simulink model "nms_model"  (Simulink 7.5)
settings: Solver=ode15s  StartTime=0.0  StopTime=60  FixedStep=1e-3  MaxStep=ts_max  RelTol=1e-3  AbsTol=1e-4
InitFcn:
  | nms_model_MechInit
  | nms_model_ControlInit
values from neighbouring files (symbols this model uses):
  c = 0.05    [muscleParams.m]    (also in nms_model_MechInit.m)
  c_jointstop = 0.3 / (pi/180)    (= 17.1887338539)    [muscleParams.m]    (also in nms_model_MechInit.m)
  D12_F = 0.16    [nms_model_MechInit.m]
  D12_S = L_S    (= 0.5)    [nms_model_MechInit.m]
  D12_T = L_T    (= 0.5)    [nms_model_MechInit.m]
  D13_F = 0.20    (= 0.2)    [nms_model_MechInit.m]
  D1G_F = 0.14    [nms_model_MechInit.m]
  D1G_HAT = 0.35    [nms_model_MechInit.m]
  D1G_S = 0.3    [nms_model_MechInit.m]
  D1G_T = 0.3    [nms_model_MechInit.m]
  DeltaThRef = 5e-3    (= 0.005)    [nms_model_MechInit.m]
  eref = 0.04    [muscleParams.m]    (also in nms_model_MechInit.m)
  FmaxGAS = 1500    [nms_model_MechInit.m]
  FmaxGLU = 1500    [nms_model_MechInit.m]
  FmaxHAM = 3000    [nms_model_MechInit.m]
  FmaxHFL = 2000    [nms_model_MechInit.m]
  FmaxSOL = 4000    [nms_model_MechInit.m]
  FmaxTA = 800    [nms_model_MechInit.m]
  FmaxVAS = 300    [muscleParams.m]    (also in nms_model_MechInit.m = 6000)
  GainDeltaTheta = 2 /100*180/pi    (= 1.14591559026)    [nms_model_ControlInit.m]
  GainGAS = 1.1/FmaxGAS    [nms_model_ControlInit.m]
  GainGLU = 0.5/FmaxGLU    [nms_model_ControlInit.m]
  GainHAM = 0.65/FmaxHAM    [nms_model_ControlInit.m]
  GainHAMHFL = 4    [nms_model_ControlInit.m]
  GainHFL = 0.5    [nms_model_ControlInit.m]
  GainKneOverExt = 2    [nms_model_ControlInit.m]
  GainSOL = 1.2/FmaxSOL    [nms_model_ControlInit.m]
  GainSOLTA = 0.4/FmaxSOL    [nms_model_ControlInit.m]
  GainTA = 1.1    [nms_model_ControlInit.m]
  GainVAS = 1.2/FmaxVAS    [nms_model_ControlInit.m]
  In_F = 0.005    [nms_model_MechInit.m]
  In_HAT = 3    [nms_model_MechInit.m]
  In_S = 0.05    [nms_model_MechInit.m]
  In_T = 0.15    [nms_model_MechInit.m]
  K = 5    [muscleParams.m]    (also in nms_model_MechInit.m)
  k_gx = (2*(m_F+m_S+m_T)+m_HAT)*g/0.1    (= 7848)    [nms_model_MechInit.m]
  k_gy = (2*(m_F+m_S+m_T)+m_HAT)*g/0.01    (= 78480)    [nms_model_MechInit.m]
  k_pressure = m_HAT * 9.81 / DeltaThRef    (= 104967)    [nms_model_MechInit.m]
  K_swing = 0.25    [nms_model_ControlInit.m]
  KneePh23Offset = 170*pi/180    (= 2.96705972839)    [nms_model_ControlInit.m]
  LceOffsetHAM = 0.85    [nms_model_ControlInit.m]
  LceOffsetHFL = 0.65    [nms_model_ControlInit.m]
  LceOffsetTA = 1-0.5*w    [nms_model_ControlInit.m]
  LongDelay = 0.020    (= 0.02)    [nms_model_ControlInit.m]
  loptGAS = 0.05    [nms_model_MechInit.m]
  loptGLU = 0.11    [nms_model_MechInit.m]
  loptHAM = 0.10    (= 0.1)    [nms_model_MechInit.m]
  loptHFL = 0.11    [nms_model_MechInit.m]
  loptSOL = 0.04    [nms_model_MechInit.m]
  loptTA = 0.06    [nms_model_MechInit.m]
  loptVAS = 0.13    [muscleParams.m]    (also in nms_model_MechInit.m = 0.08)
  lslackGAS = 0.40    (= 0.4)    [nms_model_MechInit.m]
  lslackGLU = 0.13    [nms_model_MechInit.m]
  lslackHAM = 0.31    [nms_model_MechInit.m]
  lslackHFL = 0.10    (= 0.1)    [nms_model_MechInit.m]
  lslackSOL = 0.26    [nms_model_MechInit.m]
  lslackTA = 0.24    [nms_model_MechInit.m]
  lslackVAS = 0.23    [muscleParams.m]    (also in nms_model_MechInit.m)
  m_F = 1.25    [nms_model_MechInit.m]
  m_HAT = 53.5    [nms_model_MechInit.m]
  m_S = 3.5    [nms_model_MechInit.m]
  m_T = 8.5    [nms_model_MechInit.m]
  MidDelay = 0.010    (= 0.01)    [nms_model_ControlInit.m]
  mu_slide = 0.8    [nms_model_MechInit.m]
  mu_stick = 0.9    [nms_model_MechInit.m]
  N = 1.5    [muscleParams.m]    (also in nms_model_MechInit.m)
  phi12_LowLimit = 70*pi/180    (= 1.2217304764)    [nms_model_MechInit.m]
  phi12_UpLimit = 180*pi/180    (= 3.14159265359)    [muscleParams.m]    (also in nms_model_MechInit.m = 2.26892802759)
  phi23_UpLimit = 159*pi/180    (= 2.77507351067)    [muscleParams.m]    (also in nms_model_MechInit.m = 3.05432619099)
  phi34_UpLimit = 230*pi/180    (= 4.01425727959)    [nms_model_MechInit.m]
  phimaxGASa = 110*pi/180    (= 1.91986217719)    [nms_model_MechInit.m]
  phimaxGASk = 140*pi/180    (= 2.44346095279)    [nms_model_MechInit.m]
  phimaxHAMk = 180*pi/180    (= 3.14159265359)    [nms_model_MechInit.m]
  phimaxSOL = 110*pi/180    (= 1.91986217719)    [nms_model_MechInit.m]
  phimaxTA = 80*pi/180    (= 1.3962634016)    [nms_model_MechInit.m]
  phimaxVAS = 90*pi/180    (= 1.57079632679)    [muscleParams.m]    (also in nms_model_MechInit.m = 2.87979326579)
  phirefGASa = 80*pi/180    (= 1.3962634016)    [nms_model_MechInit.m]
  phirefGASk = 165*pi/180    (= 2.87979326579)    [nms_model_MechInit.m]
  phirefGLU = 150*pi/180    (= 2.61799387799)    [nms_model_MechInit.m]
  phirefHAMh = 155*pi/180    (= 2.70526034059)    [nms_model_MechInit.m]
  phirefHAMk = 180*pi/180    (= 3.14159265359)    [nms_model_MechInit.m]
  phirefHFL = 180*pi/180    (= 3.14159265359)    [nms_model_MechInit.m]
  phirefSOL = 80*pi/180    (= 1.3962634016)    [nms_model_MechInit.m]
  phirefTA = 110*pi/180    (= 1.91986217719)    [nms_model_MechInit.m]
  phirefVAS = 60*pi/180    (= 1.0471975512)    [muscleParams.m]    (also in nms_model_MechInit.m = 2.18166156499)
  PosGainGG = 1/(30*pi/180)    (= 1.9098593171)    [nms_model_ControlInit.m]
  PreStimGAS = 0.01    [nms_model_ControlInit.m]
  PreStimGG = 0.05    [nms_model_ControlInit.m]
  PreStimGLU = 0.01    [nms_model_ControlInit.m]
  PreStimHAM = 0.01    [nms_model_ControlInit.m]
  PreStimHFL = 0.01    [nms_model_ControlInit.m]
  PreStimSOL = 0.01    [nms_model_ControlInit.m]
  PreStimTA = 0.01    [nms_model_ControlInit.m]
  PreStimVAS = 0.08    [nms_model_ControlInit.m]
  rGASa = 0.05    [nms_model_MechInit.m]
  rGASk = 0.05    [nms_model_MechInit.m]
  rGLU = 0.10    (= 0.1)    [nms_model_MechInit.m]
  rHAMh = 0.08    [nms_model_MechInit.m]
  rHAMk = 0.05    [nms_model_MechInit.m]
  rHFL = 0.10    (= 0.1)    [nms_model_MechInit.m]
  rhoGASa = 0.7    [nms_model_MechInit.m]
  rhoGASk = 0.7    [nms_model_MechInit.m]
  rhoGLU = 0.5    [nms_model_MechInit.m]
  rhoHAMh = 0.7    [nms_model_MechInit.m]
  rhoHAMk = 0.7    [nms_model_MechInit.m]
  rhoHFL = 0.5    [nms_model_MechInit.m]
  rhoSOL = 0.5    [nms_model_MechInit.m]
  rhoTA = 0.7    [nms_model_MechInit.m]
  rhoVAS = 3    [muscleParams.m]    (also in nms_model_MechInit.m = 0.7)
  rSOL = 0.05    [nms_model_MechInit.m]
  rTA = 0.04    [nms_model_MechInit.m]
  rVAS = 0.03    [muscleParams.m]    (also in nms_model_MechInit.m = 0.06)
  s = orProblemSendCommand(['LoadIKFastSolver robot Translation3D'],probid)    [init.m]
  ShortDelay = 0.005    [nms_model_ControlInit.m]
  SpeedGainGG = 0.2    [nms_model_ControlInit.m]
  tau = 0.01    [muscleParams.m]    (also in nms_model_MechInit.m)
  Theta0 = 6*pi/180    (= 0.10471975512)    [nms_model_ControlInit.m]
  ThPos = 4/5    (= 0.8)    [nms_model_MechInit.m]
  v_gx_max = 0.03    [nms_model_MechInit.m]
  v_gy_max = 0.03    [nms_model_MechInit.m]
  ... (+11 more)
undefined symbols (not defined in the file or in its folder): sgn
libraries: mblibv1 x60, simulink x22, simulink_extras x20
(part 5 of 9)

== system nms_model/Muscle Actuation Layer/R TA ==
  note: Excitation Contraction Coupling
  note: Tibialis Anterior Muscle-Tendon Dynamics
  STIM : Inport  OutDataType=sfix(16)  OutScaling=2^0
  lmtc [m] : Inport  Port=2  OutDataType=sfix(16)  OutScaling=2^0
  1 : Product  Inputs=**  OutDataType=sfix(16)  OutScaling=2^0  SaturateOnIntegerOverflow=on  InputSameDT=on  OutDataTypeStr=Inherit: Same as first input
  1/lslack : Gain  Gain=1/lslackTA  ParameterDataType=sfix(16)  ParameterScaling=2^0  OutDataType=sfix(16)  OutScaling=2^0  SaturateOnIntegerOverflow=on  OutDataTypeStr=Inherit: Same as input  ParamDataTypeStr=Inherit: Same as input
  BE force-length relation : Subsystem
  CE force-length relation : Subsystem
  CE inverse  force-velocity relation : Subsystem
  Constant : Constant  Value=lslackTA  OutDataType=sfix(16)  OutScaling=2^0
  ECC TransferFcn : simulink_extras/Additional Linear/Transfer Fcn (with initial outputs)  SystemSampleTime=-1  N=[1]  D="[tau  1]"  Y0=preA  U0=0
      settings: AttributesFormatString=pre-activation: %<Y0>
  Fmax : Gain  Gain=FmaxTA  ParameterDataType=sfix(16)  ParameterScaling=2^0  OutDataType=sfix(16)  OutScaling=2^0  SaturateOnIntegerOverflow=on  OutDataTypeStr=Inherit: Same as input  ParamDataTypeStr=Inherit: Same as input
  Fv = Fse / (A*Fce) : Product  Inputs=*/  OutDataType=sfix(16)  OutScaling=2^0  SaturateOnIntegerOverflow=on  InputSameDT=on  OutDataTypeStr=Inherit: Same as first input
  Integrator : Integrator  InitialConditionSource=external  LowerSaturationLimit=0.05
  PE force-length relation : Subsystem
  SE force-length relation : Subsystem
  Sum : Sum  Inputs=|+-  OutDataType=sfix(16)  OutScaling=2^0  SaturateOnIntegerOverflow=on  InputSameDT=on  OutDataTypeStr=Inherit: Same as first input
  Sum2 : Sum  Inputs=|-+  OutDataType=sfix(16)  OutScaling=2^0  SaturateOnIntegerOverflow=on  InputSameDT=on  OutDataTypeStr=Inherit: Same as first input
  Sum3 : Sum  OutDataType=sfix(16)  OutScaling=2^0  SaturateOnIntegerOverflow=on  InputSameDT=on  OutDataTypeStr=Inherit: Same as first input
  Sum4 : Sum  OutDataType=sfix(16)  OutScaling=2^0  SaturateOnIntegerOverflow=on  InputSameDT=on  OutDataTypeStr=Inherit: Same as first input
  lce/lopt : Gain  Gain=1/loptTA  ParameterDataType=sfix(16)  ParameterScaling=2^0  OutDataType=sfix(16)  OutScaling=2^0  SaturateOnIntegerOverflow=on  OutDataTypeStr=Inherit: Same as input  ParamDataTypeStr=Inherit: Same as input
  vmax*lopt : Gain  Gain=vmaxTA*loptTA  ParameterDataType=sfix(16)  ParameterScaling=2^0  OutDataType=sfix(16)  OutScaling=2^0  SaturateOnIntegerOverflow=on  OutDataTypeStr=Inherit: Same as input  ParamDataTypeStr=Inherit: Same as input
  Fmtc : Outport  OutDataType=sfix(16)  OutScaling=2^0  InitialOutput=0
  Lce : Outport  Port=2  OutDataType=sfix(16)  OutScaling=2^0  InitialOutput=0
  Vce : Outport  Port=3  OutDataType=sfix(16)  OutScaling=2^0  InitialOutput=0
  Lse : Outport  Port=4  OutDataType=sfix(16)  OutScaling=2^0  InitialOutput=0
  A : Outport  Port=5  OutDataType=sfix(16)  OutScaling=2^0  InitialOutput=0
  wires:
  CE inverse  force-velocity relation/1(v[vmax]) -> vmax*lopt/1
  Sum3/1 -> Fv = Fse / (A*Fce)/2
  BE force-length relation/1(fbe [Fmax]) -> Sum4/2
  1/1 -> Sum3/2
  PE force-length relation/1(fpe [Fmax]) -> Sum3/1
  Sum4/1 -> Fv = Fse / (A*Fce)/1
  CE force-length relation/1(fce [Fmax]) -> 1/1
  Constant/1 -> Sum2/1
  Sum2/1 -> Integrator/2
  SE force-length relation/1(fse [Fmax]) -> Sum4/1, Fmax/1
  1/lslack/1 -> SE force-length relation/1(lse [lslack])
  Fmax/1 -> Fmtc/1  "Fmtc"
  lmtc [m]/1 -> Sum/1, Sum2/2  "lmtc"
  vmax*lopt/1 -> Integrator/1, Vce/1  "vce"
  Fv = Fse / (A*Fce)/1 -> CE inverse  force-velocity relation/1(Fv[Fmax])  "fv"
  lce/lopt/1 -> PE force-length relation/1(lce [lopt]), BE force-length relation/1(lce [lopt]), CE force-length relation/1(lce [lopt])
  Sum/1 -> Lse/1, 1/lslack/1  "lse"
  Integrator/1 -> lce/lopt/1, Sum/2, Lce/1  "lce"
  STIM/1 -> ECC TransferFcn/1
  ECC TransferFcn/1 -> 1/2, A/1

== system nms_model/Muscle Actuation Layer/R TA Link ==
  note: Muscle Length and Moment Arm
  phi12 [rad] : Inport  OutDataType=sfix(16)  OutScaling=2^0
  Constant : Constant  Value=lslackTA+loptTA  OutDataType=sfix(16)  OutScaling=2^0
  Constant2 : Constant  Value=phirefTA  OutDataType=sfix(16)  OutScaling=2^0
  Constant3 : Constant  Value=phimaxTA  OutDataType=sfix(16)  OutScaling=2^0
  Demux : Demux  Outputs=2
  Gain2 : Gain  Gain=rTA  ParameterDataType=sfix(16)  ParameterScaling=2^0  OutDataType=sfix(16)  OutScaling=2^0
  Gain4 : Gain  Gain=rhoTA  ParameterDataType=sfix(16)  ParameterScaling=2^0  OutDataType=sfix(16)  OutScaling=2^0
  Mux : Mux  Inputs=2
  Sum2 : Sum  Inputs=|+-  OutDataType=sfix(16)  OutScaling=2^0
  Sum3 : Sum  Inputs=-+|  OutDataType=sfix(16)  OutScaling=2^0
  Sum4 : Sum  Inputs=+-  OutDataType=sfix(16)  OutScaling=2^0
  Sum5 : Sum  Inputs=|+-  OutDataType=sfix(16)  OutScaling=2^0
  length change term : Trigonometry
  offset correction term : Trigonometry
  variable lever term : Trigonometry  Operator=cos
  lmtc [m] : Outport  OutDataType=sfix(16)  OutScaling=2^0
  lever [m] : Outport  Port=2  OutDataType=sfix(16)  OutScaling=2^0
  wires:
  phi12 [rad]/1 -> Sum3/2
  Sum3/1 -> variable lever term/1, length change term/1
  Constant3/1 -> Sum3/1, Sum2/2
  Sum2/1 -> offset correction term/1
  Constant2/1 -> Sum2/1
  length change term/1 -> Sum4/2
  offset correction term/1 -> Sum4/1
  Sum4/1 -> Mux/1
  Constant/1 -> Sum5/1
  Sum5/1 -> lmtc [m]/1
  Gain4/1 -> Sum5/2
  variable lever term/1 -> Mux/2
  Mux/1 -> Gain2/1
  Gain2/1 -> Demux/1
  Demux/1 -> Gain4/1
  Demux/2 -> lever [m]/1

== system nms_model/Muscle Actuation Layer/R VAS ==
  note: VASTI Muscle-Tendon Dynamics
  note: Excitation Contraction Coupling
  STIM : Inport  OutDataType=sfix(16)  OutScaling=2^0
  lmtc [m] : Inport  Port=2  OutDataType=sfix(16)  OutScaling=2^0
  1 : Product  Inputs=**  OutDataType=sfix(16)  OutScaling=2^0  SaturateOnIntegerOverflow=on  InputSameDT=on  OutDataTypeStr=Inherit: Same as first input
  1/lslack : Gain  Gain=1/lslackVAS  ParameterDataType=sfix(16)  ParameterScaling=2^0  OutDataType=sfix(16)  OutScaling=2^0  SaturateOnIntegerOverflow=on  OutDataTypeStr=Inherit: Same as input  ParamDataTypeStr=Inherit: Same as input
  BE force-length relation : Subsystem
  CE force-length relation : Subsystem
  CE inverse  force-velocity relation : Subsystem
  Constant : Constant  Value=lslackVAS  OutDataType=sfix(16)  OutScaling=2^0
  ECC TransferFcn : simulink_extras/Additional Linear/Transfer Fcn (with initial outputs)  SystemSampleTime=-1  N=[1]  D="[tau  1]"  Y0=preA  U0=0
      settings: AttributesFormatString=pre-activation: %<Y0>
  Fmax : Gain  Gain=FmaxVAS  ParameterDataType=sfix(16)  ParameterScaling=2^0  OutDataType=sfix(16)  OutScaling=2^0  SaturateOnIntegerOverflow=on  OutDataTypeStr=Inherit: Same as input  ParamDataTypeStr=Inherit: Same as input
  Fv = Fse / (A*Fce) : Product  Inputs=*/  OutDataType=sfix(16)  OutScaling=2^0  SaturateOnIntegerOverflow=on  InputSameDT=on  OutDataTypeStr=Inherit: Same as first input
  Integrator : Integrator  InitialConditionSource=external  LowerSaturationLimit=0.05
  PE force-length relation : Subsystem
  SE force-length relation : Subsystem
  Sum : Sum  Inputs=|+-  OutDataType=sfix(16)  OutScaling=2^0  SaturateOnIntegerOverflow=on  InputSameDT=on  OutDataTypeStr=Inherit: Same as first input
  Sum2 : Sum  Inputs=|-+  OutDataType=sfix(16)  OutScaling=2^0  SaturateOnIntegerOverflow=on  InputSameDT=on  OutDataTypeStr=Inherit: Same as first input
  Sum3 : Sum  OutDataType=sfix(16)  OutScaling=2^0  SaturateOnIntegerOverflow=on  InputSameDT=on  OutDataTypeStr=Inherit: Same as first input
  Sum4 : Sum  OutDataType=sfix(16)  OutScaling=2^0  SaturateOnIntegerOverflow=on  InputSameDT=on  OutDataTypeStr=Inherit: Same as first input
  lce/lopt : Gain  Gain=1/loptVAS  ParameterDataType=sfix(16)  ParameterScaling=2^0  OutDataType=sfix(16)  OutScaling=2^0  SaturateOnIntegerOverflow=on  OutDataTypeStr=Inherit: Same as input  ParamDataTypeStr=Inherit: Same as input
  vmax*lopt : Gain  Gain=vmaxVAS*loptVAS  ParameterDataType=sfix(16)  ParameterScaling=2^0  OutDataType=sfix(16)  OutScaling=2^0  SaturateOnIntegerOverflow=on  OutDataTypeStr=Inherit: Same as input  ParamDataTypeStr=Inherit: Same as input
  Fmtc : Outport  OutDataType=sfix(16)  OutScaling=2^0  InitialOutput=0
  Lce : Outport  Port=2  OutDataType=sfix(16)  OutScaling=2^0  InitialOutput=0
  Vce : Outport  Port=3  OutDataType=sfix(16)  OutScaling=2^0  InitialOutput=0
  Lse : Outport  Port=4  OutDataType=sfix(16)  OutScaling=2^0  InitialOutput=0
  A : Outport  Port=5  OutDataType=sfix(16)  OutScaling=2^0  InitialOutput=0
  wires:
  Integrator/1 -> Sum/2, lce/lopt/1, Lce/1  "lce"
  Sum/1 -> 1/lslack/1, Lse/1  "lse"
  lce/lopt/1 -> CE force-length relation/1(lce [lopt]), BE force-length relation/1(lce [lopt]), PE force-length relation/1(lce [lopt])
  Fv = Fse / (A*Fce)/1 -> CE inverse  force-velocity relation/1(Fv[Fmax])  "fv"
  vmax*lopt/1 -> Integrator/1, Vce/1  "vce"
  lmtc [m]/1 -> Sum2/2, Sum/1  "lmtc"
  Fmax/1 -> Fmtc/1  "Fmtc"
  1/lslack/1 -> SE force-length relation/1(lse [lslack])
  SE force-length relation/1(fse [Fmax]) -> Fmax/1, Sum4/1
  Sum2/1 -> Integrator/2
  Constant/1 -> Sum2/1
  CE force-length relation/1(fce [Fmax]) -> 1/1
  Sum4/1 -> Fv = Fse / (A*Fce)/1
  PE force-length relation/1(fpe [Fmax]) -> Sum3/1
  1/1 -> Sum3/2
  BE force-length relation/1(fbe [Fmax]) -> Sum4/2
  Sum3/1 -> Fv = Fse / (A*Fce)/2
  CE inverse  force-velocity relation/1(v[vmax]) -> vmax*lopt/1
  STIM/1 -> ECC TransferFcn/1
  ECC TransferFcn/1 -> 1/2, A/1

== system nms_model/Muscle Actuation Layer/R VAS Link ==
  note: Muscle Length and Moment Arm
  phi23 [rad] : Inport  OutDataType=sfix(16)  OutScaling=2^0
  Constant : Constant  Value=lslackVAS+loptVAS  OutDataType=sfix(16)  OutScaling=2^0
  Constant2 : Constant  Value=phirefVAS  OutDataType=sfix(16)  OutScaling=2^0
  Constant3 : Constant  Value=phimaxVAS  OutDataType=sfix(16)  OutScaling=2^0
  Demux : Demux  Outputs=2
  Gain2 : Gain  Gain=rVAS  ParameterDataType=sfix(16)  ParameterScaling=2^0  OutDataType=sfix(16)  OutScaling=2^0
  Gain4 : Gain  Gain=rhoVAS  ParameterDataType=sfix(16)  ParameterScaling=2^0  OutDataType=sfix(16)  OutScaling=2^0
  Mux : Mux  Inputs=2
  Sum2 : Sum  Inputs=|+-  OutDataType=sfix(16)  OutScaling=2^0
  Sum3 : Sum  Inputs=-+|  OutDataType=sfix(16)  OutScaling=2^0
  Sum4 : Sum  Inputs=+-  OutDataType=sfix(16)  OutScaling=2^0
  Sum5 : Sum  Inputs=|++  OutDataType=sfix(16)  OutScaling=2^0
  length change term : Trigonometry
  offset correction term : Trigonometry
  variable lever term : Trigonometry  Operator=cos
  lmtu [m] : Outport  OutDataType=sfix(16)  OutScaling=2^0
  lever [m] : Outport  Port=2  OutDataType=sfix(16)  OutScaling=2^0
  wires:
  phi23 [rad]/1 -> Sum3/2
  Sum3/1 -> variable lever term/1, length change term/1
  Constant3/1 -> Sum3/1, Sum2/2
  Sum2/1 -> offset correction term/1
  Constant2/1 -> Sum2/1
  length change term/1 -> Sum4/2
  offset correction term/1 -> Sum4/1
  Sum4/1 -> Mux/1
  Constant/1 -> Sum5/1
  Sum5/1 -> lmtu [m]/1
  Gain4/1 -> Sum5/2
  variable lever term/1 -> Mux/2
  Mux/1 -> Gain2/1
  Gain2/1 -> Demux/1
  Demux/1 -> Gain4/1
  Demux/2 -> lever [m]/1

== system nms_model/Neural Control Layer/Cross Influence Detection ==
  note: right leg is leading
  note: left leg is leading
  note: Double Support Cross Influences
  LStance : Inport  OutDataType=sfix(16)  OutScaling=2^0
  RStance : Inport  Port=2  OutDataType=sfix(16)  OutScaling=2^0
  DSup ends : HitCross  HitCrossingOffset=0.5  HitCrossingDirection=falling  ZeroCross=off
  Double Support? : Logic  AllPortsSameDT=off
  Double Support?1 : Logic  AllPortsSameDT=off
  Double Support?4 : Logic  AllPortsSameDT=off
  Flight? : Logic  Operator=NOR  AllPortsSameDT=off
  LLeg starts DSup : HitCross  HitCrossingOffset=0.5  HitCrossingDirection=rising  ZeroCross=off
  Memory : Memory
  Memory3 : Memory
  RLeg starts DSup : HitCross  HitCrossingOffset=0.5  HitCrossingDirection=rising  ZeroCross=off
  S-R Flip-Flop : simulink_extras/Flip Flops/S-R Flip-Flop  SystemSampleTime=-1  initial_condition=0
  S-R Flip-Flop1 : simulink_extras/Flip Flops/S-R Flip-Flop  SystemSampleTime=-1  initial_condition=0
  Terminator1 : Terminator
  Terminator2 : Terminator
  RonL : Outport  OutDataType=sfix(16)  OutScaling=2^0
  Flight : Outport  Port=2  OutDataType=sfix(16)  OutScaling=2^0
  LonR : Outport  Port=3  OutDataType=sfix(16)  OutScaling=2^0
  wires:
  S-R Flip-Flop/2 -> Terminator1/1
  Double Support?/1 -> DSup ends/1, Double Support?1/1, Double Support?4/2
  S-R Flip-Flop/1 -> LonR/1
  S-R Flip-Flop1/2 -> Terminator2/1
  LStance/1 -> Memory3/1, Double Support?/1, Flight?/1
  RStance/1 -> Memory/1, Double Support?/2, Flight?/2
  S-R Flip-Flop1/1 -> RonL/1
  Memory/1 -> RLeg starts DSup/1
  RLeg starts DSup/1 -> Double Support?1/2
  Double Support?1/1 -> S-R Flip-Flop1/1
  Memory3/1 -> LLeg starts DSup/1
  LLeg starts DSup/1 -> Double Support?4/1
  Double Support?4/1 -> S-R Flip-Flop/1
  DSup ends/1 -> S-R Flip-Flop/2, S-R Flip-Flop1/2
  Flight?/1 -> Flight/1

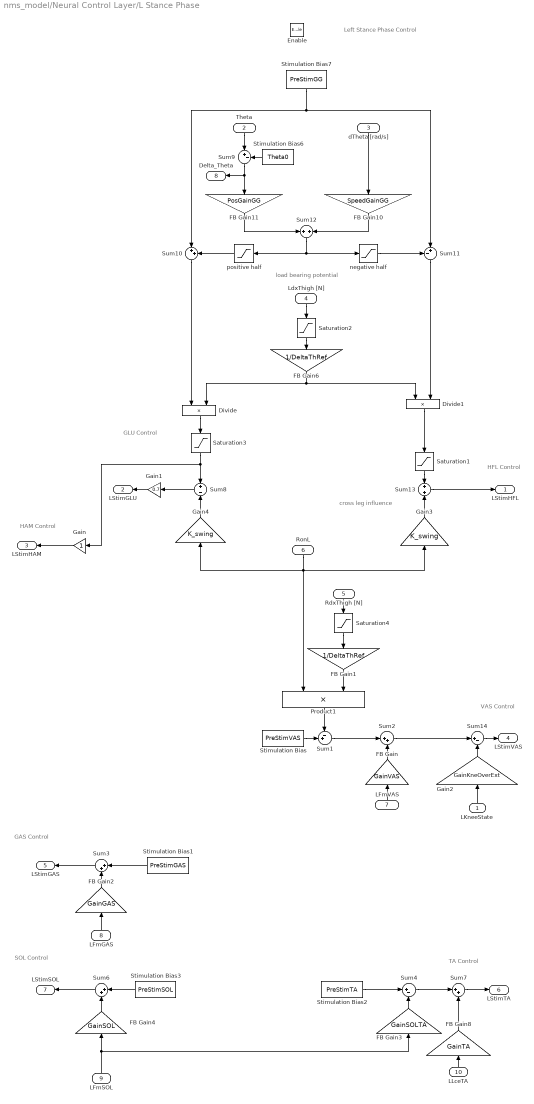
== system nms_model/Neural Control Layer/L Stance Phase ==
  note: GLU Control
  note: SOL Control
  note: TA Control
  note: GAS Control
  note: VAS Control
  note: Left Stance Phase Control
  note: HAM Control
  note: cross leg influence
  note: HFL Control
  note: load bearing potential
  LKneeState : Inport  OutDataType=sfix(16)  OutScaling=2^0
  Theta : Inport  Port=2  OutDataType=sfix(16)  OutScaling=2^0
  dTheta [rad/s] : Inport  Port=3  OutDataType=sfix(16)  OutScaling=2^0
  LdxThigh [N] : Inport  Port=4  OutDataType=sfix(16)  OutScaling=2^0
  RdxThigh [N] : Inport  Port=5  OutDataType=sfix(16)  OutScaling=2^0
  RonL : Inport  Port=6  OutDataType=sfix(16)  OutScaling=2^0
  LFmVAS : Inport  Port=7  OutDataType=sfix(16)  OutScaling=2^0
  LFmGAS : Inport  Port=8  OutDataType=sfix(16)  OutScaling=2^0
  LFmSOL : Inport  Port=9  OutDataType=sfix(16)  OutScaling=2^0
  LLceTA : Inport  Port=10  OutDataType=sfix(16)  OutScaling=2^0
  Enable : EnablePort  StatesWhenEnabling=reset
  Divide : Product  OutDataType=sfix(16)  OutScaling=2^-10
  Divide1 : Product  OutDataType=sfix(16)  OutScaling=2^-10
  FB Gain : Gain  Gain=GainVAS  ParameterDataType=sfix(16)  ParameterScaling=2^0  OutDataType=sfix(16)  OutScaling=2^0  SaturateOnIntegerOverflow=on  OutDataTypeStr=Inherit: Same as input  ParamDataTypeStr=Inherit: Same as input
  FB Gain1 : Gain  Gain=1/DeltaThRef  ParameterDataType=sfix(16)  ParameterScaling=2^0  OutDataType=sfix(16)  OutScaling=2^0  SaturateOnIntegerOverflow=on  OutDataTypeStr=Inherit: Same as input  ParamDataTypeStr=Inherit: Same as input
  FB Gain10 : Gain  Gain=SpeedGainGG  ParameterDataType=sfix(16)  ParameterScaling=2^0  OutDataType=sfix(16)  OutScaling=2^0  SaturateOnIntegerOverflow=on  OutDataTypeStr=Inherit: Same as input  ParamDataTypeStr=Inherit: Same as input
  FB Gain11 : Gain  Gain=PosGainGG  ParameterDataType=sfix(16)  ParameterScaling=2^0  OutDataType=sfix(16)  OutScaling=2^0  SaturateOnIntegerOverflow=on  OutDataTypeStr=Inherit: Same as input  ParamDataTypeStr=Inherit: Same as input
  FB Gain2 : Gain  Gain=GainGAS  ParameterDataType=sfix(16)  ParameterScaling=2^0  OutDataType=sfix(16)  OutScaling=2^0  SaturateOnIntegerOverflow=on  OutDataTypeStr=Inherit: Same as input  ParamDataTypeStr=Inherit: Same as input
  FB Gain3 : Gain  Gain=GainSOLTA  ParameterDataType=sfix(16)  ParameterScaling=2^0  OutDataType=sfix(16)  OutScaling=2^0  SaturateOnIntegerOverflow=on  OutDataTypeStr=Inherit: Same as input  ParamDataTypeStr=Inherit: Same as input
  FB Gain4 : Gain  Gain=GainSOL  ParameterDataType=sfix(16)  ParameterScaling=2^0  OutDataType=sfix(16)  OutScaling=2^0  SaturateOnIntegerOverflow=on  OutDataTypeStr=Inherit: Same as input  ParamDataTypeStr=Inherit: Same as input
  FB Gain6 : Gain  Gain=1/DeltaThRef  ParameterDataType=sfix(16)  ParameterScaling=2^0  OutDataType=sfix(16)  OutScaling=2^0  SaturateOnIntegerOverflow=on  OutDataTypeStr=Inherit: Same as input  ParamDataTypeStr=Inherit: Same as input
  FB Gain8 : Gain  Gain=GainTA  ParameterDataType=sfix(16)  ParameterScaling=2^0  OutDataType=sfix(16)  OutScaling=2^0  SaturateOnIntegerOverflow=on  OutDataTypeStr=Inherit: Same as input  ParamDataTypeStr=Inherit: Same as input
  Gain : Gain  ParameterDataType=sfix(16)  ParameterScaling=2^0  OutDataType=sfix(16)  OutScaling=2^0
  Gain1 : Gain  Gain=0.7  ParameterDataType=sfix(16)  ParameterScaling=2^0  OutDataType=sfix(16)  OutScaling=2^0
  Gain2 : Gain  Gain=GainKneOverExt  ParameterDataType=sfix(16)  ParameterScaling=2^0  OutDataType=sfix(16)  OutScaling=2^0
  Gain3 : Gain  Gain=K_swing  ParameterDataType=sfix(16)  ParameterScaling=2^0  OutDataType=sfix(16)  OutScaling=2^0
  Gain4 : Gain  Gain=K_swing  ParameterDataType=sfix(16)  ParameterScaling=2^0  OutDataType=sfix(16)  OutScaling=2^0
  Product1 : Product  OutDataType=sfix(16)  OutScaling=2^0  RndMeth=Zero
  Saturation1 : Saturate  UpperLimit=1  LowerLimit=0  ZeroCross=off
  Saturation2 : Saturate  UpperLimit=inf  LowerLimit=0  ZeroCross=off
  Saturation3 : Saturate  UpperLimit=1  LowerLimit=0  ZeroCross=off
  Saturation4 : Saturate  UpperLimit=inf  LowerLimit=0  ZeroCross=off
  Stimulation Bias : Constant  Value=PreStimVAS  OutDataType=sfix(16)  OutScaling=2^0
  Stimulation Bias1 : Constant  Value=PreStimGAS  OutDataType=sfix(16)  OutScaling=2^0
  Stimulation Bias2 : Constant  Value=PreStimTA  OutDataType=sfix(16)  OutScaling=2^0
  Stimulation Bias3 : Constant  Value=PreStimSOL  OutDataType=sfix(16)  OutScaling=2^0
  Stimulation Bias6 : Constant  Value=Theta0  OutDataType=sfix(16)  OutScaling=2^0
  Stimulation Bias7 : Constant  Value=PreStimGG  OutDataType=sfix(16)  OutScaling=2^0
  Sum1 : Sum  Inputs=-+|  OutDataType=sfix(16)  OutScaling=2^0  SaturateOnIntegerOverflow=on  InputSameDT=on  OutDataTypeStr=Inherit: Same as first input
  Sum{2..3,6..7,10} (5 alike) : Sum  Inputs=|++  OutDataType=sfix(16)  OutScaling=2^0  SaturateOnIntegerOverflow=on  InputSameDT=on  OutDataTypeStr=Inherit: Same as first input
  Sum11 : Sum  Inputs=-+|  OutDataType=sfix(16)  OutScaling=2^0  SaturateOnIntegerOverflow=on  InputSameDT=on  OutDataTypeStr=Inherit: Same as first input
  Sum12 : Sum  OutDataType=sfix(16)  OutScaling=2^0  SaturateOnIntegerOverflow=on  InputSameDT=on  OutDataTypeStr=Inherit: Same as first input
  Sum13 : Sum  OutDataType=sfix(16)  OutScaling=2^0  SaturateOnIntegerOverflow=on  InputSameDT=on  OutDataTypeStr=Inherit: Same as first input
  Sum14 : Sum  Inputs=|+-  OutDataType=sfix(16)  OutScaling=2^0  SaturateOnIntegerOverflow=on  InputSameDT=on  OutDataTypeStr=Inherit: Same as first input
  Sum4 : Sum  Inputs=|+-  OutDataType=sfix(16)  OutScaling=2^0  SaturateOnIntegerOverflow=on  InputSameDT=on  OutDataTypeStr=Inherit: Same as first input
  Sum8 : Sum  Inputs=+-  OutDataType=sfix(16)  OutScaling=2^0  SaturateOnIntegerOverflow=on  InputSameDT=on  OutDataTypeStr=Inherit: Same as first input
  Sum9 : Sum  Inputs=|+-  OutDataType=sfix(16)  OutScaling=2^0  SaturateOnIntegerOverflow=on  InputSameDT=on  OutDataTypeStr=Inherit: Same as first input
  negative half : Saturate  UpperLimit=0  LowerLimit=-inf  ZeroCross=off
  positive half : Saturate  UpperLimit=inf  LowerLimit=0  ZeroCross=off
  LStimHFL : Outport  OutDataType=sfix(16)  OutScaling=2^0  OutputWhenDisabled=reset  InitialOutput=0
  LStimGLU : Outport  Port=2  OutDataType=sfix(16)  OutScaling=2^0  OutputWhenDisabled=reset  InitialOutput=0
  LStimHAM : Outport  Port=3  OutDataType=sfix(16)  OutScaling=2^0  OutputWhenDisabled=reset  InitialOutput=0
  LStimVAS : Outport  Port=4  OutDataType=sfix(16)  OutScaling=2^0  OutputWhenDisabled=reset  InitialOutput=0
  LStimGAS : Outport  Port=5  OutDataType=sfix(16)  OutScaling=2^0  OutputWhenDisabled=reset  InitialOutput=0
  LStimTA : Outport  Port=6  OutDataType=sfix(16)  OutScaling=2^0  OutputWhenDisabled=reset  InitialOutput=0
  LStimSOL : Outport  Port=7  OutDataType=sfix(16)  OutScaling=2^0  OutputWhenDisabled=reset  InitialOutput=0
  Delta_Theta : Outport  Port=8  OutDataType=sfix(16)  OutScaling=2^0  InitialOutput=0
  wires:
  Sum1/1 -> Sum2/1
  FB Gain/1 -> Sum2/2
  FB Gain1/1 -> Product1/2
  Saturation4/1 -> FB Gain1/1
  dTheta [rad/s]/1 -> FB Gain10/1
  Stimulation Bias6/1 -> Sum9/2
  Theta/1 -> Sum9/1
  negative half/1 -> Sum11/1
  Sum9/1 -> FB Gain11/1, Delta_Theta/1
  LFmSOL/1 -> FB Gain4/1, FB Gain3/1
  LFmVAS/1 -> FB Gain/1
  RdxThigh [N]/1 -> Saturation4/1
  LFmGAS/1 -> FB Gain2/1
  FB Gain4/1 -> Sum6/2
  Sum6/1 -> LStimSOL/1
  Stimulation Bias1/1 -> Sum3/1
  Sum3/1 -> LStimGAS/1
  FB Gain2/1 -> Sum3/2
  positive half/1 -> Sum10/2
  Stimulation Bias7/1 -> Sum10/1, Sum11/2
  FB Gain11/1 -> Sum12/1
  FB Gain10/1 -> Sum12/2
  Sum12/1 -> positive half/1, negative half/1
  Sum13/1 -> LStimHFL/1
  Product1/1 -> Sum1/1
  Saturation1/1 -> Sum13/1
  Saturation2/1 -> FB Gain6/1
  Sum11/1 -> Divide1/2
  Sum10/1 -> Divide/1
  LdxThigh [N]/1 -> Saturation2/1
  Divide1/1 -> Saturation1/1
  Gain1/1 -> LStimGLU/1
  FB Gain3/1 -> Sum4/2
  Stimulation Bias2/1 -> Sum4/1
  Sum4/1 -> Sum7/1
  Sum7/1 -> LStimTA/1
  FB Gain8/1 -> Sum7/2
  LLceTA/1 -> FB Gain8/1
  Stimulation Bias/1 -> Sum1/2
  Sum2/1 -> Sum14/1
  Sum14/1 -> LStimVAS/1
  Gain3/1 -> Sum13/2
  Stimulation Bias3/1 -> Sum6/1
  FB Gain6/1 -> Divide/2, Divide1/1
  Divide/1 -> Saturation3/1
  Sum8/1 -> Gain1/1
  Gain4/1 -> Sum8/2
  Saturation3/1 -> Sum8/1, Gain/1
  Gain2/1 -> Sum14/2
  LKneeState/1 -> Gain2/1
  RonL/1 -> Product1/1, Gain3/1, Gain4/1
  Gain/1 -> LStimHAM/1

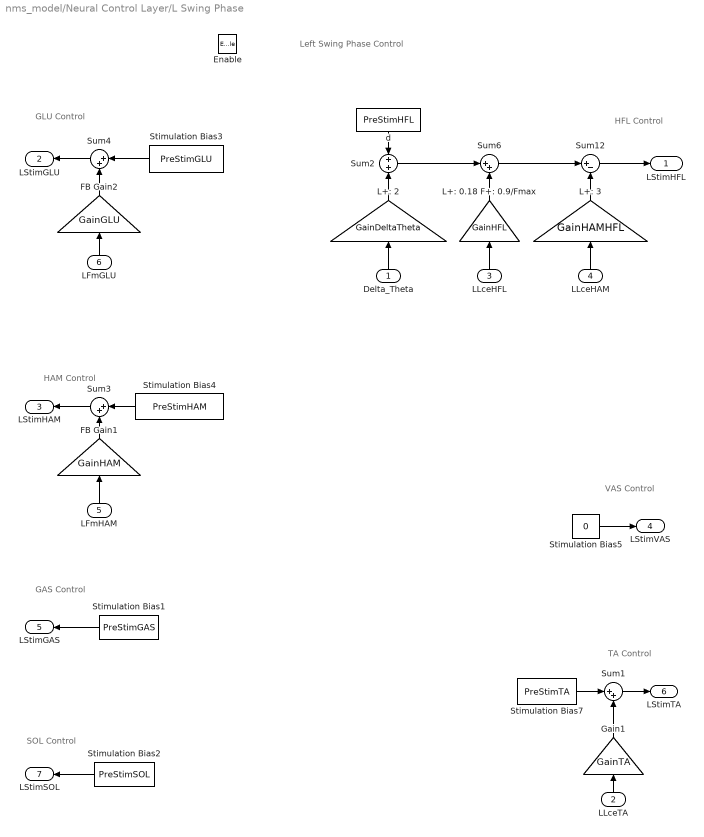
== system nms_model/Neural Control Layer/L Swing Phase ==
  note: SOL Control
  note: GAS Control
  note: VAS Control
  note: Left Swing Phase Control
  note: HAM Control
  note: GLU Control
  note: HFL Control
  note: TA Control
  Delta_Theta : Inport  OutDataType=sfix(16)  OutScaling=2^0
  LLceTA : Inport  Port=2  OutDataType=sfix(16)  OutScaling=2^0
  LLceHFL : Inport  Port=3  OutDataType=sfix(16)  OutScaling=2^0
  LLceHAM : Inport  Port=4  OutDataType=sfix(16)  OutScaling=2^0
  LFmHAM : Inport  Port=5  OutDataType=sfix(16)  OutScaling=2^0
  LFmGLU : Inport  Port=6  OutDataType=sfix(16)  OutScaling=2^0
  Enable : EnablePort  StatesWhenEnabling=reset
  FB Gain1 : Gain  Gain=GainHAM  ParameterDataType=sfix(16)  ParameterScaling=2^0  OutDataType=sfix(16)  OutScaling=2^0  SaturateOnIntegerOverflow=on  OutDataTypeStr=Inherit: Same as input  ParamDataTypeStr=Inherit: Same as input
  FB Gain2 : Gain  Gain=GainGLU  ParameterDataType=sfix(16)  ParameterScaling=2^0  OutDataType=sfix(16)  OutScaling=2^0  SaturateOnIntegerOverflow=on  OutDataTypeStr=Inherit: Same as input  ParamDataTypeStr=Inherit: Same as input
  Gain1 : Gain  Gain=GainTA  ParameterDataType=sfix(16)  ParameterScaling=2^0  OutDataType=sfix(16)  OutScaling=2^0
  L+: 0.18 F+: 0.9/Fmax : Gain  Gain=GainHFL  ParameterDataType=sfix(16)  ParameterScaling=2^0  OutDataType=sfix(16)  OutScaling=2^0  SaturateOnIntegerOverflow=on  OutDataTypeStr=Inherit: Same as input  ParamDataTypeStr=Inherit: Same as input
  L+: 2 : Gain  Gain=GainDeltaTheta  ParameterDataType=sfix(16)  ParameterScaling=2^0  OutDataType=sfix(16)  OutScaling=2^0  SaturateOnIntegerOverflow=on  OutDataTypeStr=Inherit: Same as input  ParamDataTypeStr=Inherit: Same as input
  L+: 3 : Gain  Gain=GainHAMHFL  ParameterDataType=sfix(16)  ParameterScaling=2^0  OutDataType=sfix(16)  OutScaling=2^0  SaturateOnIntegerOverflow=on  OutDataTypeStr=Inherit: Same as input  ParamDataTypeStr=Inherit: Same as input
  Stimulation Bias1 : Constant  Value=PreStimGAS  OutDataType=sfix(16)  OutScaling=2^0
  Stimulation Bias2 : Constant  Value=PreStimSOL  OutDataType=sfix(16)  OutScaling=2^0
  Stimulation Bias3 : Constant  Value=PreStimGLU  OutDataType=sfix(16)  OutScaling=2^0
  Stimulation Bias4 : Constant  Value=PreStimHAM  OutDataType=sfix(16)  OutScaling=2^0
  Stimulation Bias5 : Constant  Value=0  OutDataType=sfix(16)  OutScaling=2^0
  Stimulation Bias7 : Constant  Value=PreStimTA  OutDataType=sfix(16)  OutScaling=2^0
  Sum{1,3..4,6} (4 alike) : Sum  Inputs=|++  OutDataType=sfix(16)  OutScaling=2^0  SaturateOnIntegerOverflow=on  InputSameDT=on  OutDataTypeStr=Inherit: Same as first input
  Sum12 : Sum  Inputs=|+-  OutDataType=sfix(16)  OutScaling=2^0  SaturateOnIntegerOverflow=on  InputSameDT=on  OutDataTypeStr=Inherit: Same as first input
  Sum2 : Sum  OutDataType=sfix(16)  OutScaling=2^0  SaturateOnIntegerOverflow=on  InputSameDT=on  OutDataTypeStr=Inherit: Same as first input
  d : Constant  Value=PreStimHFL  OutDataType=sfix(16)  OutScaling=2^0
  LStimHFL : Outport  OutDataType=sfix(16)  OutScaling=2^0  OutputWhenDisabled=reset  InitialOutput=0
  LStimGLU : Outport  Port=2  OutDataType=sfix(16)  OutScaling=2^0  OutputWhenDisabled=reset  InitialOutput=0
  LStimHAM : Outport  Port=3  OutDataType=sfix(16)  OutScaling=2^0  OutputWhenDisabled=reset  InitialOutput=0
  LStimVAS : Outport  Port=4  OutDataType=sfix(16)  OutScaling=2^0  OutputWhenDisabled=reset  InitialOutput=0
  LStimGAS : Outport  Port=5  OutDataType=sfix(16)  OutScaling=2^0  OutputWhenDisabled=reset  InitialOutput=0
  LStimTA : Outport  Port=6  OutDataType=sfix(16)  OutScaling=2^0  OutputWhenDisabled=reset  InitialOutput=0
  LStimSOL : Outport  Port=7  OutDataType=sfix(16)  OutScaling=2^0  OutputWhenDisabled=reset  InitialOutput=0
  wires:
  Stimulation Bias1/1 -> LStimGAS/1
  Stimulation Bias2/1 -> LStimSOL/1
  FB Gain1/1 -> Sum3/2
  Stimulation Bias4/1 -> Sum3/1
  LLceTA/1 -> Gain1/1
  Stimulation Bias7/1 -> Sum1/1
  Sum1/1 -> LStimTA/1
  Gain1/1 -> Sum1/2
  Sum3/1 -> LStimHAM/1
  Stimulation Bias5/1 -> LStimVAS/1
  LLceHFL/1 -> L+: 0.18 F+: 0.9/Fmax/1
  L+: 0.18 F+: 0.9/Fmax/1 -> Sum6/2
  LLceHAM/1 -> L+: 3/1
  L+: 3/1 -> Sum12/2
  Sum6/1 -> Sum12/1
  Delta_Theta/1 -> L+: 2/1
  d/1 -> Sum2/1
  Sum2/1 -> Sum6/1
  L+: 2/1 -> Sum2/2
  FB Gain2/1 -> Sum4/2
  LFmGLU/1 -> FB Gain2/1
  Stimulation Bias3/1 -> Sum4/1
  Sum4/1 -> LStimGLU/1
  LFmHAM/1 -> FB Gain1/1
  Sum12/1 -> LStimHFL/1

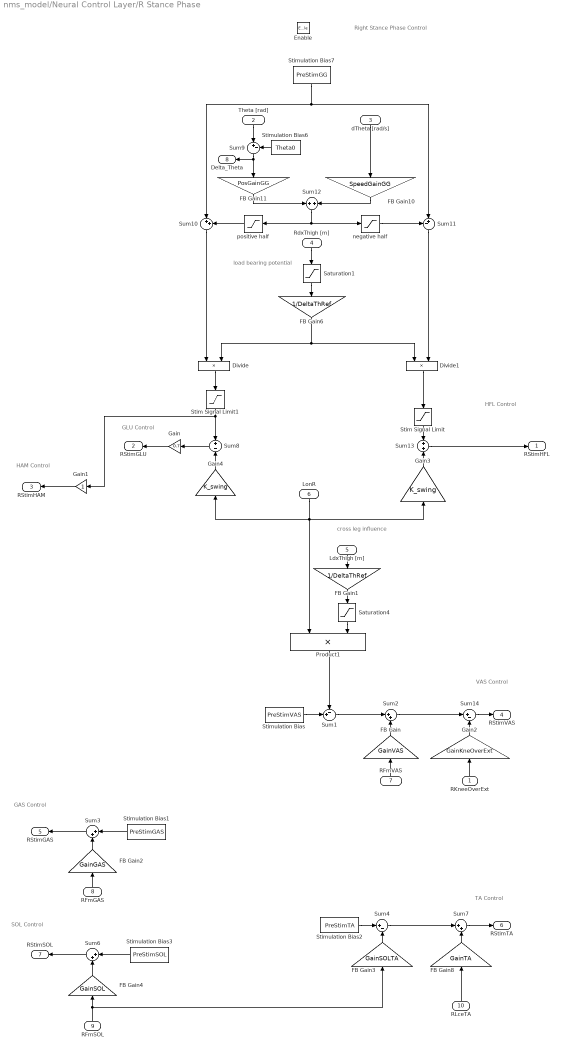
== system nms_model/Neural Control Layer/R Stance Phase ==
  note: HFL Control
  note: GLU Control
  note: SOL Control
  note: TA Control
  note: GAS Control
  note: VAS Control
  note: Right Stance Phase Control
  note: HAM Control
  note: cross leg influence
  note: load bearing potential
  RKneeOverExt : Inport  OutDataType=sfix(16)  OutScaling=2^0
  Theta [rad] : Inport  Port=2  OutDataType=sfix(16)  OutScaling=2^0
  dTheta [rad/s] : Inport  Port=3  OutDataType=sfix(16)  OutScaling=2^0
  RdxThigh [m] : Inport  Port=4  OutDataType=sfix(16)  OutScaling=2^0
  LdxThigh [m] : Inport  Port=5  OutDataType=sfix(16)  OutScaling=2^0
  LonR : Inport  Port=6  OutDataType=sfix(16)  OutScaling=2^0
  RFmVAS : Inport  Port=7  OutDataType=sfix(16)  OutScaling=2^0
  RFmGAS : Inport  Port=8  OutDataType=sfix(16)  OutScaling=2^0
  RFmSOL : Inport  Port=9  OutDataType=sfix(16)  OutScaling=2^0
  RLceTA : Inport  Port=10  OutDataType=sfix(16)  OutScaling=2^0
  Enable : EnablePort  StatesWhenEnabling=reset
  Divide : Product  OutDataType=sfix(16)  OutScaling=2^-10
  Divide1 : Product  OutDataType=sfix(16)  OutScaling=2^-10
  FB Gain : Gain  Gain=GainVAS  ParameterDataType=sfix(16)  ParameterScaling=2^0  OutDataType=sfix(16)  OutScaling=2^0  SaturateOnIntegerOverflow=on  OutDataTypeStr=Inherit: Same as input  ParamDataTypeStr=Inherit: Same as input
  FB Gain1 : Gain  Gain=1/DeltaThRef  ParameterDataType=sfix(16)  ParameterScaling=2^0  OutDataType=sfix(16)  OutScaling=2^0  SaturateOnIntegerOverflow=on  OutDataTypeStr=Inherit: Same as input  ParamDataTypeStr=Inherit: Same as input
  FB Gain10 : Gain  Gain=SpeedGainGG  ParameterDataType=sfix(16)  ParameterScaling=2^0  OutDataType=sfix(16)  OutScaling=2^0  SaturateOnIntegerOverflow=on  OutDataTypeStr=Inherit: Same as input  ParamDataTypeStr=Inherit: Same as input
  FB Gain11 : Gain  Gain=PosGainGG  ParameterDataType=sfix(16)  ParameterScaling=2^0  OutDataType=sfix(16)  OutScaling=2^0  SaturateOnIntegerOverflow=on  OutDataTypeStr=Inherit: Same as input  ParamDataTypeStr=Inherit: Same as input
  FB Gain2 : Gain  Gain=GainGAS  ParameterDataType=sfix(16)  ParameterScaling=2^0  OutDataType=sfix(16)  OutScaling=2^0  SaturateOnIntegerOverflow=on  OutDataTypeStr=Inherit: Same as input  ParamDataTypeStr=Inherit: Same as input
  FB Gain3 : Gain  Gain=GainSOLTA  ParameterDataType=sfix(16)  ParameterScaling=2^0  OutDataType=sfix(16)  OutScaling=2^0  SaturateOnIntegerOverflow=on  OutDataTypeStr=Inherit: Same as input  ParamDataTypeStr=Inherit: Same as input
  FB Gain4 : Gain  Gain=GainSOL  ParameterDataType=sfix(16)  ParameterScaling=2^0  OutDataType=sfix(16)  OutScaling=2^0  SaturateOnIntegerOverflow=on  OutDataTypeStr=Inherit: Same as input  ParamDataTypeStr=Inherit: Same as input
  FB Gain6 : Gain  Gain=1/DeltaThRef  ParameterDataType=sfix(16)  ParameterScaling=2^0  OutDataType=sfix(16)  OutScaling=2^0  SaturateOnIntegerOverflow=on  OutDataTypeStr=Inherit: Same as input  ParamDataTypeStr=Inherit: Same as input
  FB Gain8 : Gain  Gain=GainTA  ParameterDataType=sfix(16)  ParameterScaling=2^0  OutDataType=sfix(16)  OutScaling=2^0  SaturateOnIntegerOverflow=on  OutDataTypeStr=Inherit: Same as input  ParamDataTypeStr=Inherit: Same as input
  Gain : Gain  Gain=0.7  ParameterDataType=sfix(16)  ParameterScaling=2^0  OutDataType=sfix(16)  OutScaling=2^0
  Gain1 : Gain  ParameterDataType=sfix(16)  ParameterScaling=2^0  OutDataType=sfix(16)  OutScaling=2^0
  Gain2 : Gain  Gain=GainKneOverExt  ParameterDataType=sfix(16)  ParameterScaling=2^0  OutDataType=sfix(16)  OutScaling=2^0
  Gain3 : Gain  Gain=K_swing  ParameterDataType=sfix(16)  ParameterScaling=2^0  OutDataType=sfix(16)  OutScaling=2^0
  Gain4 : Gain  Gain=K_swing  ParameterDataType=sfix(16)  ParameterScaling=2^0  OutDataType=sfix(16)  OutScaling=2^0
  Product1 : Product  OutDataType=sfix(16)  OutScaling=2^0  RndMeth=Zero
  Saturation1 : Saturate  UpperLimit=inf  LowerLimit=0  ZeroCross=off
  Saturation4 : Saturate  UpperLimit=inf  LowerLimit=0  ZeroCross=off
  Stim Signal Limit : Saturate  UpperLimit=1  LowerLimit=0  ZeroCross=off
  Stim Signal Limit1 : Saturate  UpperLimit=1  LowerLimit=0  ZeroCross=off
  Stimulation Bias : Constant  Value=PreStimVAS  OutDataType=sfix(16)  OutScaling=2^0
  Stimulation Bias1 : Constant  Value=PreStimGAS  OutDataType=sfix(16)  OutScaling=2^0
  Stimulation Bias2 : Constant  Value=PreStimTA  OutDataType=sfix(16)  OutScaling=2^0
  Stimulation Bias3 : Constant  Value=PreStimSOL  OutDataType=sfix(16)  OutScaling=2^0
  Stimulation Bias6 : Constant  Value=Theta0  OutDataType=sfix(16)  OutScaling=2^0
  Stimulation Bias7 : Constant  Value=PreStimGG  OutDataType=sfix(16)  OutScaling=2^0
  Sum1 : Sum  Inputs=-+|  OutDataType=sfix(16)  OutScaling=2^0  SaturateOnIntegerOverflow=on  InputSameDT=on  OutDataTypeStr=Inherit: Same as first input
  Sum{2..3,6..7,10} (5 alike) : Sum  Inputs=|++  OutDataType=sfix(16)  OutScaling=2^0  SaturateOnIntegerOverflow=on  InputSameDT=on  OutDataTypeStr=Inherit: Same as first input
  Sum11 : Sum  Inputs=-+|  OutDataType=sfix(16)  OutScaling=2^0  SaturateOnIntegerOverflow=on  InputSameDT=on  OutDataTypeStr=Inherit: Same as first input
  Sum12 : Sum  OutDataType=sfix(16)  OutScaling=2^0  SaturateOnIntegerOverflow=on  InputSameDT=on  OutDataTypeStr=Inherit: Same as first input
  Sum13 : Sum  OutDataType=sfix(16)  OutScaling=2^0  SaturateOnIntegerOverflow=on  InputSameDT=on  OutDataTypeStr=Inherit: Same as first input
  Sum14 : Sum  Inputs=|+-  OutDataType=sfix(16)  OutScaling=2^0  SaturateOnIntegerOverflow=on  InputSameDT=on  OutDataTypeStr=Inherit: Same as first input
  Sum4 : Sum  Inputs=|+-  OutDataType=sfix(16)  OutScaling=2^0  SaturateOnIntegerOverflow=on  InputSameDT=on  OutDataTypeStr=Inherit: Same as first input
  Sum8 : Sum  Inputs=+-  OutDataType=sfix(16)  OutScaling=2^0  SaturateOnIntegerOverflow=on  InputSameDT=on  OutDataTypeStr=Inherit: Same as first input
  Sum9 : Sum  Inputs=|+-  OutDataType=sfix(16)  OutScaling=2^0  SaturateOnIntegerOverflow=on  InputSameDT=on  OutDataTypeStr=Inherit: Same as first input
  negative half : Saturate  UpperLimit=0  LowerLimit=-inf  ZeroCross=off
  positive half : Saturate  UpperLimit=inf  LowerLimit=0  ZeroCross=off
  RStimHFL : Outport  OutDataType=sfix(16)  OutScaling=2^0  OutputWhenDisabled=reset  InitialOutput=0
  RStimGLU : Outport  Port=2  OutDataType=sfix(16)  OutScaling=2^0  OutputWhenDisabled=reset  InitialOutput=0
  RStimHAM : Outport  Port=3  OutDataType=sfix(16)  OutScaling=2^0  OutputWhenDisabled=reset  InitialOutput=0
  RStimVAS : Outport  Port=4  OutDataType=sfix(16)  OutScaling=2^0  OutputWhenDisabled=reset  InitialOutput=0
  RStimGAS : Outport  Port=5  OutDataType=sfix(16)  OutScaling=2^0  OutputWhenDisabled=reset  InitialOutput=0
  RStimTA : Outport  Port=6  OutDataType=sfix(16)  OutScaling=2^0  OutputWhenDisabled=reset  InitialOutput=0
  RStimSOL : Outport  Port=7  OutDataType=sfix(16)  OutScaling=2^0  OutputWhenDisabled=reset  InitialOutput=0
  Delta_Theta : Outport  Port=8  OutDataType=sfix(16)  OutScaling=2^0  InitialOutput=0
  wires:
  Saturation4/1 -> Product1/2
  dTheta [rad/s]/1 -> FB Gain10/1
  Stimulation Bias6/1 -> Sum9/2
  Theta [rad]/1 -> Sum9/1
  negative half/1 -> Sum11/1
  Sum9/1 -> FB Gain11/1, Delta_Theta/1
  RFmSOL/1 -> FB Gain4/1, FB Gain3/1
  RFmVAS/1 -> FB Gain/1
  LdxThigh [m]/1 -> FB Gain1/1
  RFmGAS/1 -> FB Gain2/1
  FB Gain4/1 -> Sum6/2
  Sum6/1 -> RStimSOL/1
  FB Gain3/1 -> Sum4/2
  Stimulation Bias2/1 -> Sum4/1
  Sum3/1 -> RStimGAS/1
  FB Gain2/1 -> Sum3/2
  positive half/1 -> Sum10/2
  Stimulation Bias7/1 -> Sum10/1, Sum11/2
  FB Gain11/1 -> Sum12/1
  FB Gain10/1 -> Sum12/2
  Sum12/1 -> positive half/1, negative half/1
  Sum13/1 -> RStimHFL/1
  Product1/1 -> Sum1/1
  Stim Signal Limit/1 -> Sum13/1
  RdxThigh [m]/1 -> Saturation1/1
  Sum10/1 -> Divide/1
  Sum11/1 -> Divide1/2
  Saturation1/1 -> FB Gain6/1
  Divide1/1 -> Stim Signal Limit/1
  FB Gain/1 -> Sum2/2
  Sum4/1 -> Sum7/1
  Sum7/1 -> RStimTA/1
  RLceTA/1 -> FB Gain8/1
  FB Gain8/1 -> Sum7/2
  RKneeOverExt/1 -> Gain2/1
  Sum14/1 -> RStimVAS/1
  Gain/1 -> RStimGLU/1
  Stimulation Bias3/1 -> Sum6/1
  Stimulation Bias1/1 -> Sum3/1
  Gain3/1 -> Sum13/2
  FB Gain6/1 -> Divide/2, Divide1/1
  Divide/1 -> Stim Signal Limit1/1
  Stim Signal Limit1/1 -> Sum8/1, Gain1/1
  Stimulation Bias/1 -> Sum1/2
  Sum1/1 -> Sum2/1
  Sum2/1 -> Sum14/1
  Gain2/1 -> Sum14/2
  Gain4/1 -> Sum8/2
  Sum8/1 -> Gain/1
  LonR/1 -> Product1/1, Gain3/1, Gain4/1
  FB Gain1/1 -> Saturation4/1
  Gain1/1 -> RStimHAM/1

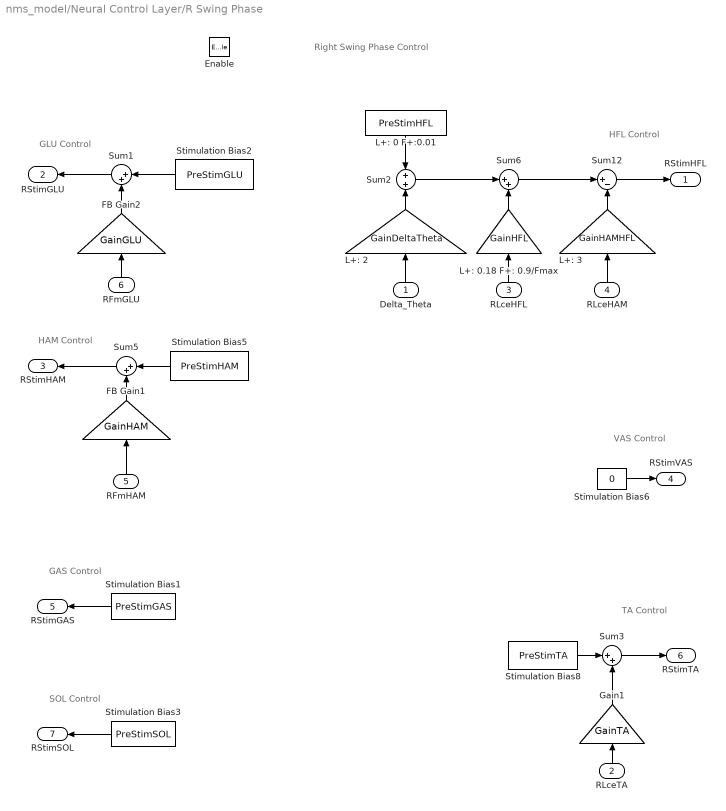
== system nms_model/Neural Control Layer/R Swing Phase ==
  note: Right Swing Phase Control
  note: VAS Control
  note: GAS Control
  note: TA Control
  note: SOL Control
  note: GLU Control
  note: HFL Control
  note: HAM Control
  Delta_Theta : Inport  OutDataType=sfix(16)  OutScaling=2^0
  RLceTA : Inport  Port=2  OutDataType=sfix(16)  OutScaling=2^0
  RLceHFL : Inport  Port=3  OutDataType=sfix(16)  OutScaling=2^0
  RLceHAM : Inport  Port=4  OutDataType=sfix(16)  OutScaling=2^0
  RFmHAM : Inport  Port=5  OutDataType=sfix(16)  OutScaling=2^0
  RFmGLU : Inport  Port=6  OutDataType=sfix(16)  OutScaling=2^0
  Enable : EnablePort  StatesWhenEnabling=reset
  FB Gain1 : Gain  Gain=GainHAM  ParameterDataType=sfix(16)  ParameterScaling=2^0  OutDataType=sfix(16)  OutScaling=2^0  SaturateOnIntegerOverflow=on  OutDataTypeStr=Inherit: Same as input  ParamDataTypeStr=Inherit: Same as input
  FB Gain2 : Gain  Gain=GainGLU  ParameterDataType=sfix(16)  ParameterScaling=2^0  OutDataType=sfix(16)  OutScaling=2^0  SaturateOnIntegerOverflow=on  OutDataTypeStr=Inherit: Same as input  ParamDataTypeStr=Inherit: Same as input
  Gain1 : Gain  Gain=GainTA  ParameterDataType=sfix(16)  ParameterScaling=2^0  OutDataType=sfix(16)  OutScaling=2^0
  L+: 0 F+:0.01 : Constant  Value=PreStimHFL  OutDataType=sfix(16)  OutScaling=2^0
  L+: 0.18 F+: 0.9/Fmax : Gain  Gain=GainHFL  ParameterDataType=sfix(16)  ParameterScaling=2^0  OutDataType=sfix(16)  OutScaling=2^0  SaturateOnIntegerOverflow=on  OutDataTypeStr=Inherit: Same as input  ParamDataTypeStr=Inherit: Same as input
  L+: 2 : Gain  Gain=GainDeltaTheta  ParameterDataType=sfix(16)  ParameterScaling=2^0  OutDataType=sfix(16)  OutScaling=2^0  SaturateOnIntegerOverflow=on  OutDataTypeStr=Inherit: Same as input  ParamDataTypeStr=Inherit: Same as input
  L+: 3 : Gain  Gain=GainHAMHFL  ParameterDataType=sfix(16)  ParameterScaling=2^0  OutDataType=sfix(16)  OutScaling=2^0  SaturateOnIntegerOverflow=on  OutDataTypeStr=Inherit: Same as input  ParamDataTypeStr=Inherit: Same as input
  Stimulation Bias1 : Constant  Value=PreStimGAS  OutDataType=sfix(16)  OutScaling=2^0
  Stimulation Bias2 : Constant  Value=PreStimGLU  OutDataType=sfix(16)  OutScaling=2^0
  Stimulation Bias3 : Constant  Value=PreStimSOL  OutDataType=sfix(16)  OutScaling=2^0
  Stimulation Bias5 : Constant  Value=PreStimHAM  OutDataType=sfix(16)  OutScaling=2^0
  Stimulation Bias6 : Constant  Value=0  OutDataType=sfix(16)  OutScaling=2^0
  Stimulation Bias8 : Constant  Value=PreStimTA  OutDataType=sfix(16)  OutScaling=2^0
  Sum{1,3,5..6} (4 alike) : Sum  Inputs=|++  OutDataType=sfix(16)  OutScaling=2^0  SaturateOnIntegerOverflow=on  InputSameDT=on  OutDataTypeStr=Inherit: Same as first input
  Sum12 : Sum  Inputs=|+-  OutDataType=sfix(16)  OutScaling=2^0  SaturateOnIntegerOverflow=on  InputSameDT=on  OutDataTypeStr=Inherit: Same as first input
  Sum2 : Sum  OutDataType=sfix(16)  OutScaling=2^0  SaturateOnIntegerOverflow=on  InputSameDT=on  OutDataTypeStr=Inherit: Same as first input
  RStimHFL : Outport  OutDataType=sfix(16)  OutScaling=2^0  OutputWhenDisabled=reset  InitialOutput=0
  RStimGLU : Outport  Port=2  OutDataType=sfix(16)  OutScaling=2^0  OutputWhenDisabled=reset  InitialOutput=0
  RStimHAM : Outport  Port=3  OutDataType=sfix(16)  OutScaling=2^0  OutputWhenDisabled=reset  InitialOutput=0
  RStimVAS : Outport  Port=4  OutDataType=sfix(16)  OutScaling=2^0  OutputWhenDisabled=reset  InitialOutput=0
  RStimGAS : Outport  Port=5  OutDataType=sfix(16)  OutScaling=2^0  OutputWhenDisabled=reset  InitialOutput=0
  RStimTA : Outport  Port=6  OutDataType=sfix(16)  OutScaling=2^0  OutputWhenDisabled=reset  InitialOutput=0
  RStimSOL : Outport  Port=7  OutDataType=sfix(16)  OutScaling=2^0  OutputWhenDisabled=reset  InitialOutput=0
  wires:
  Stimulation Bias1/1 -> RStimGAS/1
  Stimulation Bias3/1 -> RStimSOL/1
  FB Gain1/1 -> Sum5/2
  Stimulation Bias5/1 -> Sum5/1
  RLceTA/1 -> Gain1/1
  Stimulation Bias8/1 -> Sum3/1
  Sum3/1 -> RStimTA/1
  Gain1/1 -> Sum3/2
  Sum5/1 -> RStimHAM/1
  Stimulation Bias6/1 -> RStimVAS/1
  L+: 0.18 F+: 0.9/Fmax/1 -> Sum6/2
  RLceHAM/1 -> L+: 3/1
  Sum6/1 -> Sum12/1
  RLceHFL/1 -> L+: 0.18 F+: 0.9/Fmax/1
  L+: 0 F+:0.01/1 -> Sum2/1
  Sum2/1 -> Sum6/1
  L+: 2/1 -> Sum2/2
  Delta_Theta/1 -> L+: 2/1
  L+: 3/1 -> Sum12/2
  FB Gain2/1 -> Sum1/2
  RFmGLU/1 -> FB Gain2/1
  Stimulation Bias2/1 -> Sum1/1
  Sum1/1 -> RStimGLU/1
  RFmHAM/1 -> FB Gain1/1
  Sum12/1 -> RStimHFL/1

== system nms_model/Body Mechanics Layer/Left Ball Contact/Ground Friction Model ==
  note: Horizontal Ground Friction Model
  note: Vertical Ground Stiction Model
  dy [m] : Inport  OutDataType=sfix(16)  OutScaling=2^0
  vy [m/s] : Inport  Port=2  OutDataType=sfix(16)  OutScaling=2^0
  x [m] : Inport  Port=3  OutDataType=sfix(16)  OutScaling=2^0
  vx [m/s] : Inport  Port=4  OutDataType=sfix(16)  OutScaling=2^0
  Contact! : EnablePort  StatesWhenEnabling=reset
  Data Type Conversion : DataTypeConversion  OutDataTypeMode=double  OutDataType=sfix(16)  OutScaling=2^0  OutDataTypeStr=double
  Friction Switch : Subsystem
  Gain3 : Gain  Gain=k_gy  ParameterDataType=sfix(16)  ParameterScaling=2^0  OutDataType=sfix(16)  OutScaling=2^0
  Gain4 : Gain  Gain=1/v_gy_max  ParameterDataType=sfix(16)  ParameterScaling=2^0  OutDataType=sfix(16)  OutScaling=2^0
  Logical Operator : Logic  Operator=NOT  AllPortsSameDT=off  OutDataTypeMode=boolean  OutDataTypeStr=boolean
  Mux1 : Mux  Inputs=2
  Sum1 : Sum  OutDataType=sfix(16)  OutScaling=2^0
  X-Axis Kinetic Friction Model : Subsystem
  X-Axis Static Friction Model : Subsystem
  Y-Axis Ground Force : Fcn  Expr="- u(1)  *  (1-u(2)) * (u(2)<1)"
  Fy_Ground[N] : Outport  OutDataType=sfix(16)  OutScaling=2^0  OutputWhenDisabled=reset  InitialOutput=0
      settings: AttributesFormatString=initial = '%<InitialOutput>'\nwhen disabled = '%<OutputWhenDisabled>'
  Fx_Friction [N] : Outport  Port=2  OutDataType=sfix(16)  OutScaling=2^0  OutputWhenDisabled=reset  InitialOutput=0
      settings: AttributesFormatString=initial = '%<InitialOutput>'\nwhen\ndisabled\n'%<OutputWhenDisabled>'
  Stiction! : Outport  Port=3  OutDataType=sfix(16)  OutScaling=2^0  OutputWhenDisabled=reset  InitialOutput=0
      settings: AttributesFormatString=initial = '%<InitialOutput>'\nwhen\ndisabled\n'%<OutputWhenDisabled>'
  wires:
  dy [m]/1 -> Gain3/1
  vy [m/s]/1 -> Gain4/1
  x [m]/1 -> X-Axis Static Friction Model/2(pos [m]), X-Axis Kinetic Friction Model/1(pos [m])
  vx [m/s]/1 -> X-Axis Static Friction Model/3(vel [m/s]), X-Axis Kinetic Friction Model/2(vel [m/s])
  X-Axis Kinetic Friction Model/1(posFP [m]) -> X-Axis Static Friction Model/4(posFP [m])
  X-Axis Kinetic Friction Model/3(F_Slide [N]) -> Sum1/2
  X-Axis Static Friction Model/1(F_Stick [N]) -> Sum1/1
  Sum1/1 -> Fx_Friction [N]/1
  Friction Switch/1(Stiction) -> X-Axis Static Friction Model/Enable, Logical Operator/1, Data Type Conversion/1
  X-Axis Static Friction Model/2(Sliding!) -> Friction Switch/1(Slide!)
  X-Axis Kinetic Friction Model/2(Stiction!) -> Friction Switch/2(Stick!)
  Logical Operator/1 -> X-Axis Kinetic Friction Model/Enable
  Data Type Conversion/1 -> Stiction!/1
  Mux1/1 -> Y-Axis Ground Force/1
  Gain3/1 -> Mux1/1
  Gain4/1 -> Mux1/2
  Y-Axis Ground Force/1 -> Fy_Ground[N]/1, X-Axis Static Friction Model/1(F_Normal [N]), X-Axis Kinetic Friction Model/3(F_Normal [N])
